simulink library "gbt_library"  (Simulink 7.4)
settings: Solver=ode45  StartTime=0.0  StopTime=10.0  RelTol=1e-3
undefined symbols (not defined in the file or in its folder): xlipgetpartsetting
libraries: xbsIndex_r4 x1348, casper_library_misc x29, casper_library_flow_control x4
(part 11 of 11)

== system gbt_library/half_band_filter_xblock/parallel_fir3/f0/fir_col1/fir_tap1 ==
  a : Inport
  b : Inport  Port=2
  Constant : xbsIndex_r4/Constant  arith_type=Signed (2's comp)  const=4  n_bits=25  bin_pt=24  explicit_period=on  period=1  equ=P=C  opselect=C  inp2=PCIN>>17  opr=+  inp1=P  carry=CIN  dbl_ovrd=off  block_type=constant
      settings: block_version=11.4
  Mult : xbsIndex_r4/Mult  precision=Full  arith_type="Signed  (2's comp)"  n_bits=18  bin_pt=17  quantization=Truncate  overflow=Wrap  en=off  latency=1  dbl_ovrd=off  use_behavioral_HDL=on  opt=Speed  use_embedded=on  optimum_pipeline=off  pipeline=on  use_rpm=off  placement_style=Rectangular shape  block_type=mult
      settings: block_version=11.4
  Mult1 : xbsIndex_r4/Mult  precision=Full  arith_type="Signed  (2's comp)"  n_bits=18  bin_pt=17  quantization=Truncate  overflow=Wrap  en=off  latency=1  dbl_ovrd=off  use_behavioral_HDL=on  opt=Speed  use_embedded=on  optimum_pipeline=off  pipeline=on  use_rpm=off  placement_style=Rectangular shape  block_type=mult
      settings: block_version=11.4
  Register : xbsIndex_r4/Register  init=0  rst=off  en=off  dbl_ovrd=off  block_type=register
      settings: block_version=11.4
  Register1 : xbsIndex_r4/Register  init=0  rst=off  en=off  dbl_ovrd=off  block_type=register
      settings: block_version=11.4
  a_out : Outport
  b_out : Outport  Port=2
  real : Outport  Port=3
  imag : Outport  Port=4
  wires:
  Constant/1 -> Mult1/1, Mult/1
  b/1 -> Register1/1, Mult/2
  a/1 -> Register/1, Mult1/2
  Register1/1 -> b_out/1
  Register/1 -> a_out/1
  Mult1/1 -> real/1
  Mult/1 -> imag/1
